simulink model "oLDI_exc"  (R2019b)
settings: Solver=FixedStepAuto  StartTime=0.0  StopTime=110  FixedStep=1e-3  RelTol=1e-3
values from neighbouring files (symbols this model uses):
  l = 100e-6    (= 0.0001)    [oLDI_main_Vdd.m]    (also in oLDI_main_Vtau.m)
libraries: fl_lib x19, nesl_utility x6
settings Model: Creator=M.J. Mir  LastModifiedBy=yeeyoung
settings SolverCC: ZeroCrossAlgorithm=Adaptive
settings SFSimCC: CustomCodeUndefinedFunction=UseInterfaceOnly

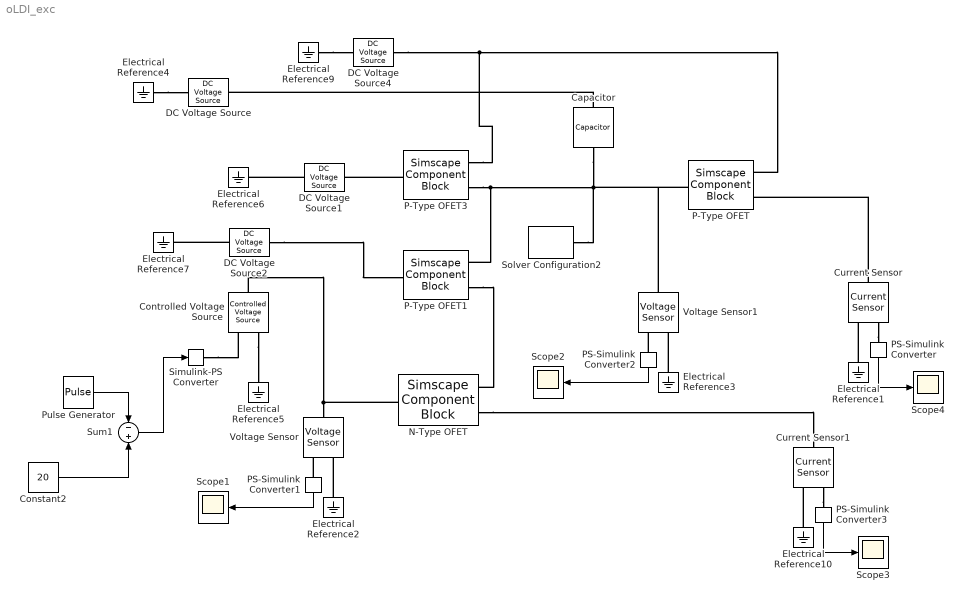
== system oLDI_exc ==
  Capacitor : fl_lib/Electrical/Electrical Elements/Capacitor  c=Csyn nF  r=0 Ohm  g=0 1/Ohm  i_specify=off  i_priority=None  i=0 A  i_nominal_specify=off  i_nominal_unit=A  i_nominal_value=1  v_specify=off  v_priority=None  v=0 V  v_nominal_specify=off  v_nominal_unit=V  v_nominal_value=1  vc_specify=off  vc_priority=High  vc=0 V  vc_nominal_specify=off  vc_nominal_unit=V  vc_nominal_value=1
  Constant2 : Constant  Value=20
  Controlled Voltage Source : fl_lib/Electrical/Electrical Sources/Controlled Voltage Source
  Current Sensor : fl_lib/Electrical/Electrical Sensors/Current Sensor
  Current Sensor1 : fl_lib/Electrical/Electrical Sensors/Current Sensor
  DC Voltage Source : fl_lib/Electrical/Electrical Sources/DC Voltage Source  v0=Vdd V
  DC Voltage Source1 : fl_lib/Electrical/Electrical Sources/DC Voltage Source  v0=Vtau V
  DC Voltage Source2 : fl_lib/Electrical/Electrical Sources/DC Voltage Source  v0=Vw V
  DC Voltage Source4 : fl_lib/Electrical/Electrical Sources/DC Voltage Source  v0=Vdd V
  Electrical Reference{1..7,9..10} (9 alike) : fl_lib/Electrical/Electrical Elements/Electrical Reference
  N-Type OFET : SimscapeComponentBlock  SourceFile=N_Marinov_OFET  ComponentPath=N_Marinov_OFET  ComponentVariants=N_Marinov_OFET  ComponentVariantNames=N_Marinov_OFET  ClassName=N_Marinov_OFET  SchemaVersion=1  Gamma=gama_n  Lambda=landa_n  Vbb=Vbb_n  Vss=Vss_n  aaa=aaa_n  bbb=bbb_n  ccc=ccc_n  Mu0=mu0_n  Vt=Vt_n V  Cox=ci  W=W_n  L=l  i_specify=off  i_priority=None  i=0 A  i_nominal_specify=off  i_nominal_unit=A  i_nominal_value=1  Vgs_specify=off  Vgs_priority=None  Vgs=0 V  Vgs_nominal_specify=off  Vgs_nominal_unit=V  Vgs_nominal_value=1  Vds_specify=off  Vds_priority=None  Vds=0 V  Vds_nominal_specify=off  Vds_nominal_unit=V  Vds_nominal_value=1
      settings: CopyFcn=simscape.engine.sli.internal.componentblockcallback(gcbh,'COPY')  PreCopyFcn=simscape.engine.sli.internal.componentblockcallback(gcbh,'PRECOPY')  PreDeleteFcn=simscape.engine.sli.internal.componentblockcallback(gcbh,'PREDELETE')  InternalSimscapePortConfiguration="{\"Bottom\":[],\"Left\":[{\"id\":\"g\",\"label\":\"Gate\",\"type\":\"foundation.electrical.electrical\"}],\"Right\":[{\"id\":\"d\",\"label\":\"Drain\",\"type\":\"foundation.electrical.electrical\"},{\"id\":\"s\",\"label\":\"Source\",\"type\":\"foundation.electrical.electrical\"}],\"Top\":[]}"
      mask Type: Marinov OFET
  P-Type OFET : SimscapeComponentBlock  SourceFile=P_Marinov_OFET  ComponentPath=P_Marinov_OFET  ComponentVariants=P_Marinov_OFET  ComponentVariantNames=P_Marinov_OFET  ClassName=P_Marinov_OFET  SchemaVersion=1  Gamma=gama_p  Lambda=landa_p  Vbb=Vbb_p  Vss=Vss_p  aaa=aaa_p  bbb=bbb_p  ccc=ccc_p  Mu0=mu0_p  Vt=Vt_p V  Cox=ci  W=W_p  L=l  i_specify=off  i_priority=None  i=0 A  i_nominal_specify=off  i_nominal_unit=A  i_nominal_value=1  Vsg_specify=off  Vsg_priority=None  Vsg=0 V  Vsg_nominal_specify=off  Vsg_nominal_unit=V  Vsg_nominal_value=1  Vsd_specify=off  Vsd_priority=None  Vsd=0 V  Vsd_nominal_specify=off  Vsd_nominal_unit=V  Vsd_nominal_value=1
      settings: CopyFcn=simscape.engine.sli.internal.componentblockcallback(gcbh,'COPY')  PreCopyFcn=simscape.engine.sli.internal.componentblockcallback(gcbh,'PRECOPY')  PreDeleteFcn=simscape.engine.sli.internal.componentblockcallback(gcbh,'PREDELETE')  InternalSimscapePortConfiguration="{\"Bottom\":[],\"Left\":[{\"id\":\"g\",\"label\":\"Gate\",\"type\":\"foundation.electrical.electrical\"}],\"Right\":[{\"id\":\"s\",\"label\":\"Source\",\"type\":\"foundation.electrical.electrical\"},{\"id\":\"d\",\"label\":\"Drain\",\"type\":\"foundation.electrical.electrical\"}],\"Top\":[]}"
      mask Type: Marinov OFET
  P-Type OFET1 : SimscapeComponentBlock  SourceFile=P_Marinov_OFET  ComponentPath=P_Marinov_OFET  ComponentVariants=P_Marinov_OFET  ComponentVariantNames=P_Marinov_OFET  ClassName=P_Marinov_OFET  SchemaVersion=1  Gamma=gama_p  Lambda=landa_p  Vbb=Vbb_p  Vss=Vss_p  aaa=aaa_p  bbb=bbb_p  ccc=ccc_p  Mu0=mu0_p  Vt=Vt_p V  Cox=ci  W=W_p  L=l  i_specify=off  i_priority=None  i=0 A  i_nominal_specify=off  i_nominal_unit=A  i_nominal_value=1  Vsg_specify=off  Vsg_priority=None  Vsg=0 V  Vsg_nominal_specify=off  Vsg_nominal_unit=V  Vsg_nominal_value=1  Vsd_specify=off  Vsd_priority=None  Vsd=0 V  Vsd_nominal_specify=off  Vsd_nominal_unit=V  Vsd_nominal_value=1
      settings: CopyFcn=simscape.engine.sli.internal.componentblockcallback(gcbh,'COPY')  PreCopyFcn=simscape.engine.sli.internal.componentblockcallback(gcbh,'PRECOPY')  PreDeleteFcn=simscape.engine.sli.internal.componentblockcallback(gcbh,'PREDELETE')  InternalSimscapePortConfiguration="{\"Bottom\":[],\"Left\":[{\"id\":\"g\",\"label\":\"Gate\",\"type\":\"foundation.electrical.electrical\"}],\"Right\":[{\"id\":\"s\",\"label\":\"Source\",\"type\":\"foundation.electrical.electrical\"},{\"id\":\"d\",\"label\":\"Drain\",\"type\":\"foundation.electrical.electrical\"}],\"Top\":[]}"
      mask Type: Marinov OFET
  P-Type OFET3 : SimscapeComponentBlock  SourceFile=P_Marinov_OFET  ComponentPath=P_Marinov_OFET  ComponentVariants=P_Marinov_OFET  ComponentVariantNames=P_Marinov_OFET  ClassName=P_Marinov_OFET  SchemaVersion=1  Gamma=gama_p  Lambda=landa_p  Vbb=Vbb_p  Vss=Vss_p  aaa=aaa_p  bbb=bbb_p  ccc=ccc_p  Mu0=mu0_p  Vt=Vt_p V  Cox=ci  W=W_p  L=l  i_specify=off  i_priority=None  i=0 A  i_nominal_specify=off  i_nominal_unit=A  i_nominal_value=1  Vsg_specify=off  Vsg_priority=None  Vsg=0 V  Vsg_nominal_specify=off  Vsg_nominal_unit=V  Vsg_nominal_value=1  Vsd_specify=off  Vsd_priority=None  Vsd=0 V  Vsd_nominal_specify=off  Vsd_nominal_unit=V  Vsd_nominal_value=1
      settings: CopyFcn=simscape.engine.sli.internal.componentblockcallback(gcbh,'COPY')  PreCopyFcn=simscape.engine.sli.internal.componentblockcallback(gcbh,'PRECOPY')  PreDeleteFcn=simscape.engine.sli.internal.componentblockcallback(gcbh,'PREDELETE')  InternalSimscapePortConfiguration="{\"Bottom\":[],\"Left\":[{\"id\":\"g\",\"label\":\"Gate\",\"type\":\"foundation.electrical.electrical\"}],\"Right\":[{\"id\":\"s\",\"label\":\"Source\",\"type\":\"foundation.electrical.electrical\"},{\"id\":\"d\",\"label\":\"Drain\",\"type\":\"foundation.electrical.electrical\"}],\"Top\":[]}"
      mask Type: Marinov OFET
  PS-Simulink Converter{,1..3} (4 alike) : nesl_utility/PS-Simulink Converter  PhysicalDomain=network_engine_domain  SubClassName=ps_output  LeftPortType=input  RightPortType=output  PseudoPeriodic=off  Frequencies=[]  Unit=1  AffineConversion=off
  Pulse Generator : DiscretePulseGenerator  PulseType=Time based  Amplitude=40  Period=10.1  PulseWidth=50
  Scope{1..4} (4 alike) : Scope
  Simulink-PS Converter : nesl_utility/Simulink-PS Converter  PhysicalDomain=network_engine_domain  SubClassName=ps_input  LeftPortType=input  RightPortType=output  PseudoPeriodic=off  Frequencies=[]  NoiseDistribution=none  NoiseParameters=[]  Unit=1  AffineConversion=off  FilteringAndDerivatives=provide  SimscapeFilterOrder=1  InputFilterTimeConstant=0.001  UdotUserProvided=0
  Solver Configuration2 : nesl_utility/Solver Configuration  PhysicalDomain=network_engine_domain  SubClassName=solver  LeftPortType=input  RightPortType=generic  Tones=[]  Harmonics=[]  SimulateNoise=off  Profile=off  UseLocalSampling=off  EnableSwitchedLinearOptims=on  FrequencyDomain=off  UseCCode=off  RelTol=0.001  AbsTol=1e-06  MinStep=1e-09  ToWorkspace=off  RevertToSquareIcSolve=off  NumHomotopyIterations=100  PhasorMode=off  PhasorModeNumHarmonics=1  DoDC=off  ResidualTolerance=1e-9  UseLocalSolver=off  LocalSolverChoice=NE_BACKWARD_EULER_ADVANCER  LocalSolverSampleTime=0.0001  DoFixedCost=off  MaxNonlinIter=1000  MaxModeIter=2  LinearAlgebra=auto  EquationFormulation=NE_TIME_EF  DelaysMemoryBudget=1024  AutomaticFiltering=off  FilteringTimeConstant=0.001  PartitionStorageMethod=AS_NEEDED  PartitionMemoryBudget=1024  PartitionMethod=ROBUST
  Sum1 : Sum  Inputs=-+
  Voltage Sensor : fl_lib/Electrical/Electrical Sensors/Voltage Sensor
  Voltage Sensor1 : fl_lib/Electrical/Electrical Sensors/Voltage Sensor
  wires:
  PS-Simulink Converter/1 -> Scope4/1
  PS-Simulink Converter1/1 -> Scope1/1
  PS-Simulink Converter2/1 -> Scope2/1
  Sum1/1 -> Simulink-PS Converter/1
  PS-Simulink Converter3/1 -> Scope3/1
  Pulse Generator/1 -> Sum1/1
  Constant2/1 -> Sum1/2
  connections:
  Capacitor/RConn1 -- DC Voltage Source/LConn1
  PS-Simulink Converter1/LConn1 -- Voltage Sensor/RConn1
  Current Sensor/RConn1 -- PS-Simulink Converter/LConn1
  Electrical Reference2/LConn1 -- Voltage Sensor/RConn2
  Electrical Reference1/LConn1 -- Current Sensor/RConn2
  Electrical Reference4/LConn1 -- DC Voltage Source/RConn1
  P-Type OFET3/RConn2 -- Voltage Sensor1/LConn1 -- P-Type OFET/LConn1 -- Solver Configuration2/RConn1 -- Capacitor/LConn1 -- P-Type OFET1/RConn1
  Controlled Voltage Source/RConn2 -- Electrical Reference5/LConn1
  Current Sensor/LConn1 -- P-Type OFET/RConn2
  Controlled Voltage Source/LConn1 -- N-Type OFET/LConn1 -- Voltage Sensor/LConn1
  Simulink-PS Converter/RConn1 -- Controlled Voltage Source/RConn1
  P-Type OFET3/LConn1 -- DC Voltage Source1/LConn1
  P-Type OFET1/RConn2 -- N-Type OFET/RConn1
  Electrical Reference3/LConn1 -- Voltage Sensor1/RConn2
  PS-Simulink Converter2/LConn1 -- Voltage Sensor1/RConn1
  Electrical Reference9/LConn1 -- DC Voltage Source4/RConn1
  DC Voltage Source4/LConn1 -- P-Type OFET3/RConn1 -- P-Type OFET/RConn1
  DC Voltage Source1/RConn1 -- Electrical Reference6/LConn1
  Electrical Reference10/LConn1 -- Current Sensor1/RConn2
  Current Sensor1/RConn1 -- PS-Simulink Converter3/LConn1
  N-Type OFET/RConn2 -- Current Sensor1/LConn1
  DC Voltage Source2/LConn1 -- P-Type OFET1/LConn1
  DC Voltage Source2/RConn1 -- Electrical Reference7/LConn1
